simulink model "ROS_00"  (R2022b)
settings: Solver=FixedStepAuto  StartTime=0.0  StopTime=inf  FixedStep=0.01  RelTol=1e-3
model workspace (MAT data in the model file):
  SL_ROS_VariableLengthArrays_MaxSizes.CommonInfo.ArrayTruncateAction = 'EmitWarning'
  SL_ROS_VariableLengthArrays_MaxSizes.MsgTypeMap = containers.Map
  SL_ROS_VariableLengthArrays_MaxSizes.MsgTypeMap.serialization.keys = {'sensor_msgs/CompressedImage', 'sensor_msgs/LaserScan', 'std_msgs/Int8MultiArray'}
  SL_ROS_VariableLengthArrays_MaxSizes.MsgTypeMap.serialization.values{1}(1).PropertyName = 'Data'
  SL_ROS_VariableLengthArrays_MaxSizes.MsgTypeMap.serialization.values{1}(1).DataType = 'uint8'
  SL_ROS_VariableLengthArrays_MaxSizes.MsgTypeMap.serialization.values{1}(1).MaxLength = 83420
  SL_ROS_VariableLengthArrays_MaxSizes.MsgTypeMap.serialization.values{1}(2).PropertyName = 'Format'
  SL_ROS_VariableLengthArrays_MaxSizes.MsgTypeMap.serialization.values{1}(2).DataType = 'uint8'
  SL_ROS_VariableLengthArrays_MaxSizes.MsgTypeMap.serialization.values{1}(2).MaxLength = 8
  SL_ROS_VariableLengthArrays_MaxSizes.MsgTypeMap.serialization.values{2}(1).PropertyName = 'Intensities'
  SL_ROS_VariableLengthArrays_MaxSizes.MsgTypeMap.serialization.values{2}(1).DataType = 'single'
  SL_ROS_VariableLengthArrays_MaxSizes.MsgTypeMap.serialization.values{2}(1).MaxLength = 360
  SL_ROS_VariableLengthArrays_MaxSizes.MsgTypeMap.serialization.values{2}(2).PropertyName = 'Ranges'
  SL_ROS_VariableLengthArrays_MaxSizes.MsgTypeMap.serialization.values{2}(2).DataType = 'single'
  SL_ROS_VariableLengthArrays_MaxSizes.MsgTypeMap.serialization.values{2}(2).MaxLength = 360
  SL_ROS_VariableLengthArrays_MaxSizes.MsgTypeMap.serialization.values{3}.PropertyName = 'Data'
  SL_ROS_VariableLengthArrays_MaxSizes.MsgTypeMap.serialization.values{3}.DataType = 'int8'
  SL_ROS_VariableLengthArrays_MaxSizes.MsgTypeMap.serialization.values{3}.MaxLength = 2
  SL_ROS_VariableLengthArrays_MaxSizes.MsgTypeMap.serialization.uniformity = 0
  SL_ROS_VariableLengthArrays_MaxSizes.MsgTypeMap.serialization.keyType = 'char'
  SL_ROS_VariableLengthArrays_MaxSizes.MsgTypeMap.serialization.valueType = 'any'
undefined symbols (not defined in the file): Data, Data_SL_Info, X, Y
libraries: robotlib x12
settings Model: Creator=mustacchim  LastModifiedBy=mustacchim
settings OptimizationCC: EnhancedBackFolding=on  PassReuseOutputArgsAs=Individual arguments  ZeroExternalMemoryAtStartup=off  ZeroInternalMemoryAtStartup=off  MaxStackSize=64  OptimizeBlockOrder=speed  DifferentSizesBufferReuse=on  OptimizationCustomize=off  EfficientTunableParamExpr=on
settings DebuggingCC: ParameterTunabilityLossMsg=error
settings HardwareCC: ProdBitPerPointer=32  ProdBitPerSizeT=32  ProdBitPerPtrDiffT=32  ProdLargestAtomicFloat=None  ProdIntDivRoundTo=Undefined  ProdEndianess=Unspecified  ProdWordSize=32  ProdHWDeviceType=Generic->Unspecified (assume 32-bit Generic)
settings SFSimCC: MATLABDynamicMemAlloc=off
settings RTWCC: Description=Embedded Coder  SystemTargetFile=ert.tlc  HardwareBoard=Robot Operating System (ROS)  TLCOptions="-aInlineSetEventsForThisBaseRateFcn=TLC_FALSE -aSuppressMultiTaskScheduler=TLC_FALSE  -aRateBasedStepFcn=0"  TemplateMakefile=ert_default_tmf  Toolchain=Catkin  TargetLang=C++
settings CodeAppCC: ForceParamTrailComments=on  IgnoreCustomStorageClasses=off  OperatorAnnotations=on  SimulinkDataObjDesc=on  SFDataObjDesc=on  InsertBlockDesc=on

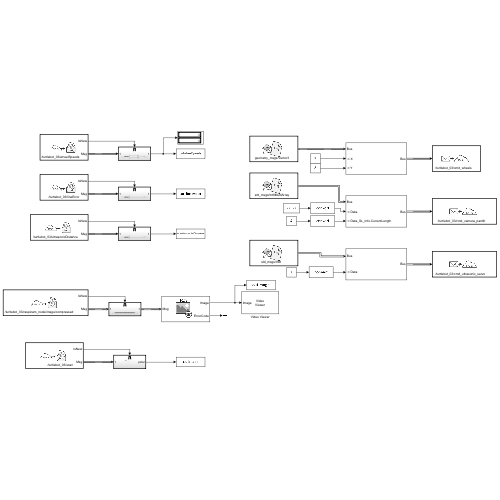
[thumbnail: Simulink's stored preview of the top-level diagram]
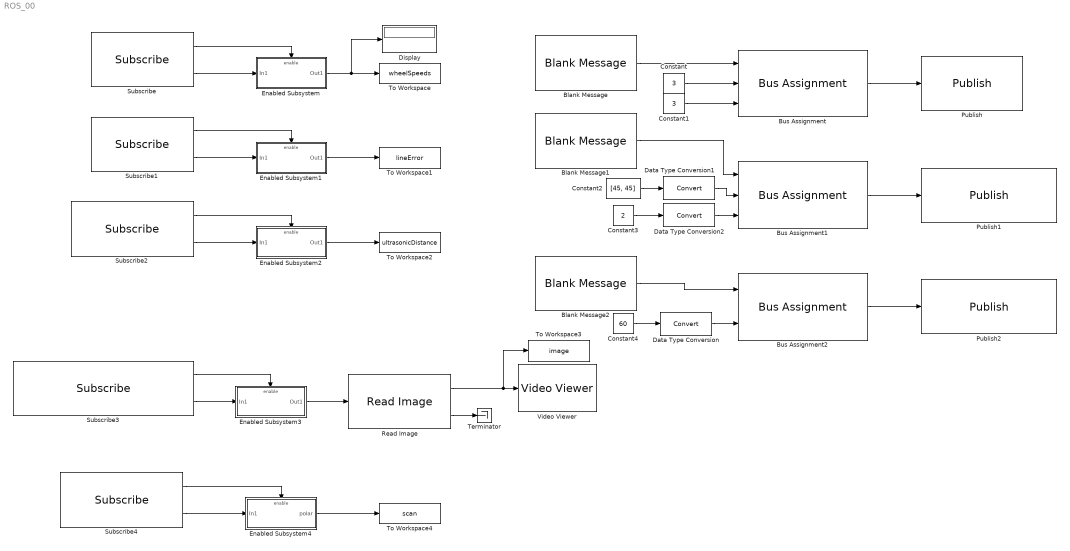
== system ROS_00 ==
  Blank Message : robotlib/Blank Message  messageClass=Message  entityType=geometry_msgs/Vector3  messageType=geometry_msgs/Vector3  SampleTime=-1  legacyBusStruct=off
      settings: LibrarySourceBlock=roslib/ROS/Blank Message
  Blank Message1 : robotlib/Blank Message  messageClass=Message  entityType=std_msgs/Int8MultiArray  messageType=std_msgs/Int8MultiArray  SampleTime=-1  legacyBusStruct=off
      settings: LibrarySourceBlock=roslib/ROS/Blank Message
  Blank Message2 : robotlib/Blank Message  messageClass=Message  entityType=std_msgs/Int8  messageType=std_msgs/Int8  SampleTime=-1  legacyBusStruct=off
      settings: LibrarySourceBlock=roslib/ROS/Blank Message
  Bus Assignment : BusAssignment  AssignedSignals=X,Y
  Bus Assignment1 : BusAssignment  AssignedSignals=Data,Data_SL_Info.CurrentLength
  Bus Assignment2 : BusAssignment  AssignedSignals=Data
  Constant : Constant  Value=3
  Constant1 : Constant  Value=3
  Constant2 : Constant  Value=[45, 45]
  Constant3 : Constant  Value=2
  Constant4 : Constant  Value=60
  Data Type Conversion : DataTypeConversion  SaturateOnIntegerOverflow=off  RndMeth=Floor
  Data Type Conversion1 : DataTypeConversion  SaturateOnIntegerOverflow=off  RndMeth=Floor
  Data Type Conversion2 : DataTypeConversion  SaturateOnIntegerOverflow=off  RndMeth=Floor
  Display : Display
  Enabled Subsystem : Subsystem  TreatAsAtomicUnit=on
  Enabled Subsystem1 : Subsystem  TreatAsAtomicUnit=on
  Enabled Subsystem2 : Subsystem  TreatAsAtomicUnit=on
  Enabled Subsystem3 : Subsystem  TreatAsAtomicUnit=on
  Enabled Subsystem4 : Subsystem  TreatAsAtomicUnit=on
  Publish : robotlib/Publish  topicSource=Select from ROS network  topic=/turtlebot_03/cmd_wheels  messageType=geometry_msgs/Vector3  legacyBusStruct=off  messageQueueLength=1
      settings: LibrarySourceBlock=roslib/ROS/Publish
  Publish1 : robotlib/Publish  topicSource=Select from ROS network  topic=/turtlebot_03/cmd_camera_pantilt  messageType=std_msgs/Int8MultiArray  legacyBusStruct=off  messageQueueLength=1
      settings: LibrarySourceBlock=roslib/ROS/Publish
  Publish2 : robotlib/Publish  topicSource=Select from ROS network  topic=/turtlebot_03/cmd_ultrasonic_servo  messageType=std_msgs/Int8  legacyBusStruct=off  messageQueueLength=1
      settings: LibrarySourceBlock=roslib/ROS/Publish
  Read Image : robotlib/Read Image  MaximumImageSize=[308, 410]  ImageEncoding=bgr8  ShowAlphaOutput=off  ShowErrorCodeOutput=on  VariableSizeOutputs=off
      settings: LibrarySourceBlock=roslib/ROS/Read Image
  Subscribe : robotlib/Subscribe  topicSource=Select from ROS network  topic=/turtlebot_03/wheelSpeeds  messageType=geometry_msgs/Vector3  SampleTime=0.02  legacyBusStruct=off  messageQueueLength=1
      settings: LibrarySourceBlock=roslib/ROS/Subscribe
  Subscribe1 : robotlib/Subscribe  topicSource=Select from ROS network  topic=/turtlebot_03/lineError  messageType=std_msgs/Float32  SampleTime=0.12  legacyBusStruct=off  messageQueueLength=1
      settings: LibrarySourceBlock=roslib/ROS/Subscribe
  Subscribe2 : robotlib/Subscribe  topicSource=Select from ROS network  topic=/turtlebot_03/ultrasonicDistance  messageType=std_msgs/Float32  SampleTime=0.11  legacyBusStruct=off  messageQueueLength=1
      settings: LibrarySourceBlock=roslib/ROS/Subscribe
  Subscribe3 : robotlib/Subscribe  topicSource=Select from ROS network  topic=/turtlebot_03/raspicam_node/image/compressed  messageType=sensor_msgs/CompressedImage  SampleTime=0.03  legacyBusStruct=off  messageQueueLength=1
      settings: LibrarySourceBlock=roslib/ROS/Subscribe
  Subscribe4 : robotlib/Subscribe  topicSource=Select from ROS network  topic=/turtlebot_03/scan  messageType=sensor_msgs/LaserScan  SampleTime=0.11  legacyBusStruct=off  messageQueueLength=1
      settings: LibrarySourceBlock=roslib/ROS/Subscribe
  Terminator : Terminator
  To Workspace : ToWorkspace  VariableName=wheelSpeeds  SaveFormat=Structure With Time  SampleTime=-1
  To Workspace1 : ToWorkspace  VariableName=lineError  SaveFormat=Structure With Time  SampleTime=-1
  To Workspace2 : ToWorkspace  VariableName=ultrasonicDistance  SaveFormat=Structure With Time  SampleTime=-1
  To Workspace3 : ToWorkspace  VariableName=image  SaveFormat=Structure With Time  SampleTime=-1
  To Workspace4 : ToWorkspace  VariableName=scan  SaveFormat=Structure With Time  SampleTime=-1
  Video Viewer : VideoViewer  FigPos=[1133 863 418 317]
  wires:
  Subscribe/1 -> Enabled Subsystem/Enable
  Subscribe/2 -> Enabled Subsystem/1(In1)
  Enabled Subsystem/1(Out1) -> Display/1, To Workspace/1
  Blank Message/1 -> Bus Assignment/1
  Constant1/1 -> Bus Assignment/3
  Constant/1 -> Bus Assignment/2
  Bus Assignment/1 -> Publish/1
  Enabled Subsystem1/1(Out1) -> To Workspace1/1
  Subscribe1/2 -> Enabled Subsystem1/1(In1)
  Enabled Subsystem2/1(Out1) -> To Workspace2/1
  Subscribe2/2 -> Enabled Subsystem2/1(In1)
  Subscribe2/1 -> Enabled Subsystem2/Enable
  Subscribe1/1 -> Enabled Subsystem1/Enable
  Blank Message1/1 -> Bus Assignment1/1
  Bus Assignment1/1 -> Publish1/1
  Blank Message2/1 -> Bus Assignment2/1
  Bus Assignment2/1 -> Publish2/1
  Constant4/1 -> Data Type Conversion/1
  Data Type Conversion/1 -> Bus Assignment2/2
  Data Type Conversion1/1 -> Bus Assignment1/2
  Constant2/1 -> Data Type Conversion1/1
  Enabled Subsystem3/1(Out1) -> Read Image/1
  Subscribe3/2 -> Enabled Subsystem3/1(In1)
  Subscribe3/1 -> Enabled Subsystem3/Enable
  Read Image/1 -> Video Viewer/1, To Workspace3/1
  Read Image/2 -> Terminator/1
  Data Type Conversion2/1 -> Bus Assignment1/3
  Constant3/1 -> Data Type Conversion2/1
  Subscribe4/2 -> Enabled Subsystem4/1(In1)
  Subscribe4/1 -> Enabled Subsystem4/Enable
  Enabled Subsystem4/1(polar) -> To Workspace4/1

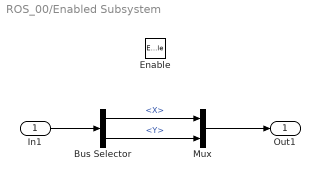
== system ROS_00/Enabled Subsystem ==
  In1 : Inport
  Enable : EnablePort
  Bus Selector : BusSelector  OutputSignals=X,Y
  Mux : Mux  Inputs=2
  Out1 : Outport
  wires:
  Mux/1 -> Out1/1
  Bus Selector/1 -> Mux/1  "<X>"
  Bus Selector/2 -> Mux/2  "<Y>"
  In1/1 -> Bus Selector/1

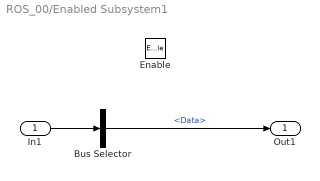
== system ROS_00/Enabled Subsystem1 ==
  In1 : Inport
  Enable : EnablePort
  Bus Selector : BusSelector  OutputSignals=Data
  Out1 : Outport
  wires:
  Bus Selector/1 -> Out1/1  "<Data>"
  In1/1 -> Bus Selector/1

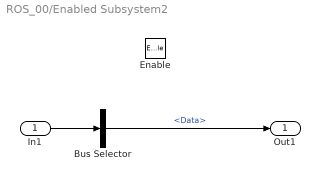
== system ROS_00/Enabled Subsystem2 ==
  In1 : Inport
  Enable : EnablePort
  Bus Selector : BusSelector  OutputSignals=Data
  Out1 : Outport
  wires:
  Bus Selector/1 -> Out1/1  "<Data>"
  In1/1 -> Bus Selector/1

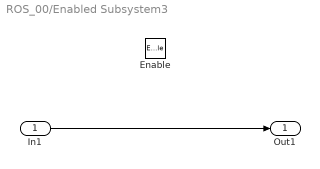
== system ROS_00/Enabled Subsystem3 ==
  In1 : Inport
  Enable : EnablePort
  Out1 : Outport
  wires:
  In1/1 -> Out1/1

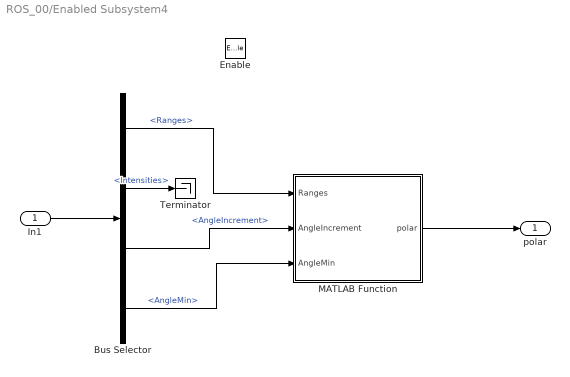
== system ROS_00/Enabled Subsystem4 ==
  In1 : Inport
  Enable : EnablePort
  Bus Selector : BusSelector  OutputSignals=Ranges,Intensities,AngleIncrement,AngleMin
  MATLAB Function : MATLAB Function  TreatAsAtomicUnit=on
  Terminator : Terminator
  polar : Outport
  wires:
  Bus Selector/1 -> MATLAB Function/1(Ranges)  "<Ranges>"
  In1/1 -> Bus Selector/1
  Bus Selector/4 -> MATLAB Function/3(AngleMin)  "<AngleMin>"
  Bus Selector/3 -> MATLAB Function/2(AngleIncrement)  "<AngleIncrement>"
  Bus Selector/2 -> Terminator/1  "<Intensities>"
  MATLAB Function/1(polar) -> polar/1

== matlab function ROS_00/Enabled Subsystem4/MATLAB Function ==
  data: Ranges input; polar output; AngleIncrement input; AngleMin input
function polar = fcn(Ranges, AngleIncrement, AngleMin)

    polar = zeros(length(Ranges), 2);
    for i = 1:length(Ranges)
        polar(i,1) = Ranges(i);
        polar(i,2) = AngleMin + ((i-1) * AngleIncrement);
    end

end
